simulink model "SkidSteeringControl"  (Simulink 8.9)
settings: Solver=VariableStepAuto  StartTime=0.0  StopTime=100  MaxStep=0.01  RelTol=1e-3
PreLoadFcn:
  | % Vehicle parameters
  | m = 1000;  % Vehicle mass
  | fR = 0.3;  % Front wheel radius
  | rR = 0.3;  % Rear wheel radius
  | J_front = 0.5;  % Front wheel moment of inertia
  | J_rear = 0.5;  % Rear wheel moment of inertia
  | J_engine = 0.01; % Engine moment of inertia
  | trans_ratio = 2.0;  % Transmission gear ratio
  | drive_ratio = 2.0;  % Final drive gear ratio
  | h = 0.5;   % Vehicle CG height above ground
  | 
  | % Aerodynamic load
  | cw = 0.34;  % Drag coefficient
  | rho = 1.18; % Air density
  | A_f = 1;    % Frontal area
  | 
  | 
  | %tire parameters
  | radiusWheel = 16*2.54/100;
  | inertiaLateral = 25*(radiusWheel)^2;
  | tireStiffness = 200000;
  | tireDamping = 1000;
StopFcn:
  | %%
  | close all;
  | figure;plot(disp_x,disp_y);grid on;axis('tight');
  | title('Vehicle Displacement Plot');
  | xlabel('Displacement X(m)');ylabel('Displacement Y(m)');
  | %%
  | figure;
  | subplot(2,1,1);
  | plot(desired_speedFL.time, desired_speedFL.signals.values,'g');grid on;hold on;
  | plot(desired_speedFR.time, desired_speedFR.signals.values,'b');grid on;
  | title('Desired Wheel Speed');
  | legend('Wheel Speed FL','Wheel Speed FR');
  | subplot(2,1,2);
  | plot(ref_speedFL.time, ref_speedFL.signals.values,'g');grid on;hold on;
  | plot(ref_speedFR.time, ref_speedFR.signals.values,'b');grid on;
  | title('Reference Wheel Speed(Slip Compensated)');
  | legend('Wheel Speed FL','Wheel Speed FR');
  | %%
  | figure;plot(yaw_rate.time,yaw_rate.signals.values);grid on;
  | title('Vehicle Yaw Rate');
  | xlabel('time(s)');ylabel('Yaw Rate(rad/s)');
  | %%
  | figure;
  | subplot(2,1,1);
  | plot(slip_WheelFL.time, slip_WheelFL.signals.values);grid on;
  | title('Wheel Slip Front Left');
  | xlabel('time(s)');ylabel('Slip Ratio');
  | subplot(2,1,2);
  | plot(slip_WheelFR.time, slip_WheelFR.signals.values);grid on;
  | title('Wheel Slip Front Right');
  | xlabel('time(s)');ylabel('Slip Ratio');
  | %%
  | figure;
  | subplot(2,1,1);
  | plot(torque_WheelFL.time, torque_WheelFL.signals.values);grid on;
  | title('Wheel Torque Front Left');
  | xlabel('time(s)');ylabel('Torque(Nm)');
  | subplot(2,1,2);
  | plot(torque_WheelFR.time, torque_WheelFR.signals.values);grid on;
  | title('Wheel Torque Front Right');
  | xlabel('time(s)');ylabel('Torque(Nm)');
libraries: nesl_utility x8, fl_lib x4, sdl_lib x4, simulink_extras x2, simulink x1
(part 2 of 2)

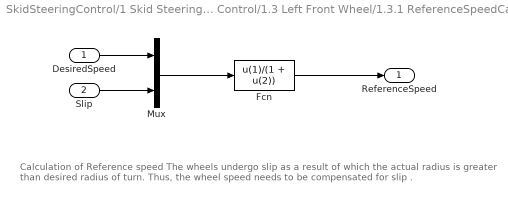
== system SkidSteeringControl/1 Skid Steering Control/1.3 Left Front Wheel/1.3.1 ReferenceSpeedCalcFR ==
  note: Calculation of Reference speed
      | The wheels undergo slip as a result of which the actual radius is greater than desired radius of turn.
      | Thus, the wheel speed needs to be compensated for slip
      | .
  DesiredSpeed : Inport
  "Slip " : Inport  Port=2
  Fcn : Fcn  Expr=u(1)/(1 + u(2))
  Mux : Mux  Inputs=2
  ReferenceSpeed : Outport
  wires:
  "Slip "/1 -> Mux/2
  Fcn/1 -> ReferenceSpeed/1
  DesiredSpeed/1 -> Mux/1
  Mux/1 -> Fcn/1

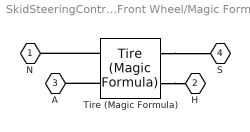
== system SkidSteeringControl/1 Skid Steering Control/1.3 Left Front Wheel/Magic Formula ==
  Tire (Magic Formula) : sdl_lib/Tires & Vehicles/Tire (Magic Formula)  parameterization=1  F_z1=3000 N  F_x1=3500 N  kappa1=10  B_m=10  C_m=1.9  D_m=1  E_m=0.97  fz0=4e+3 N  p_Cx=1.685  p_Dx=[ 1.21 -0.037 ]  p_Ex=[ 0.344 0.095 -0.02 0 ]  p_Kx=[ 21.51 -0.163 0.245 ]  p_Hx=[ -0.002 0.002 ]  p_Vx=[ 0 0 ]  v_tr_thr=0.1 m/s  r_e=radiusWheel m  model_compliance=1  stiffness=tireStiffness N/m  damping=tireDamping N/(m/s)  model_inertia=1  inertia=inertiaLateral/2 kg*m^2  initial_velocity=0 rpm  model_resistance=1  resistance_model=1  coeff=0.015  p_tire=250e3 Pa  alpha=-0.003  beta=0.97  coeff_a=84e-4  coeff_b=6.2e-4 s/m  coeff_c=1.6e-4 s^2/m^2  v_thr=1e-3 m/s
      settings: SourceProductName=Simscape Driveline
  N : PMIOPort  Port=1  Side=Left
  H : PMIOPort  Port=2  Side=Left
  A : PMIOPort  Port=3  Side=Left
  S : PMIOPort  Port=4  Side=Right
  connections:
  Tire (Magic Formula)/LConn2 -- A/RConn1
  Tire (Magic Formula)/LConn1 -- N/RConn1
  Tire (Magic Formula)/RConn2 -- H/RConn1
  Tire (Magic Formula)/RConn1 -- S/RConn1

== system SkidSteeringControl/1 Skid Steering Control/1.3 Left Front Wheel/SlipOut ==
  PS-Simulink Converter : nesl_utility/PS-Simulink Converter  PhysicalDomain=network_engine_domain  SubClassName=ps_output  LeftPortType=input  RightPortType=output  PseudoPeriodic=off  Frequencies=[]  Unit=1  AffineConversion=off
  S : PMIOPort  Port=1  Side=Left
  Slip : Outport
  wires:
  PS-Simulink Converter/1 -> Slip/1
  connections:
  S/RConn1 -- PS-Simulink Converter/LConn1

== system SkidSteeringControl/1 Skid Steering Control/1.4 Right Front Wheel/1.4.1 ReferenceSpeedCalcFR ==
  note: Calculation of Reference speed
      | The wheels undergo slip as a result of which the actual radius is greater than desired radius of turn.
      | Thus, the wheel speed needs to be compensated for slip
      | .
  DesiredSpeed : Inport
  "Slip " : Inport  Port=2
  Fcn : Fcn  Expr=u(1)/(1 + u(2))
  Mux : Mux  Inputs=2
  ReferenceSpeed : Outport
  wires:
  "Slip "/1 -> Mux/2
  Fcn/1 -> ReferenceSpeed/1
  DesiredSpeed/1 -> Mux/1
  Mux/1 -> Fcn/1

== system SkidSteeringControl/1 Skid Steering Control/1.4 Right Front Wheel/Magic Formula ==
  Tire (Magic Formula) : sdl_lib/Tires & Vehicles/Tire (Magic Formula)  parameterization=1  F_z1=3000 N  F_x1=3500 N  kappa1=10  B_m=10  C_m=1.9  D_m=1  E_m=0.97  fz0=4e+3 N  p_Cx=1.685  p_Dx=[ 1.21 -0.037 ]  p_Ex=[ 0.344 0.095 -0.02 0 ]  p_Kx=[ 21.51 -0.163 0.245 ]  p_Hx=[ -0.002 0.002 ]  p_Vx=[ 0 0 ]  v_tr_thr=0.1 m/s  r_e=radiusWheel m  model_compliance=1  stiffness=tireStiffness N/m  damping=tireDamping N/(m/s)  model_inertia=1  inertia=inertiaLateral/2 kg*m^2  initial_velocity=0 rpm  model_resistance=1  resistance_model=1  coeff=0.015  p_tire=250e3 Pa  alpha=-0.003  beta=0.97  coeff_a=84e-4  coeff_b=6.2e-4 s/m  coeff_c=1.6e-4 s^2/m^2  v_thr=1e-3 m/s
      settings: SourceProductName=Simscape Driveline
  N : PMIOPort  Port=1  Side=Left
  H : PMIOPort  Port=2  Side=Left
  A : PMIOPort  Port=3  Side=Left
  S : PMIOPort  Port=4  Side=Right
  connections:
  Tire (Magic Formula)/LConn2 -- A/RConn1
  Tire (Magic Formula)/LConn1 -- N/RConn1
  Tire (Magic Formula)/RConn2 -- H/RConn1
  Tire (Magic Formula)/RConn1 -- S/RConn1

== system SkidSteeringControl/1 Skid Steering Control/1.4 Right Front Wheel/SlipOut ==
  PS-Simulink Converter : nesl_utility/PS-Simulink Converter  PhysicalDomain=network_engine_domain  SubClassName=ps_output  LeftPortType=input  RightPortType=output  PseudoPeriodic=off  Frequencies=[]  Unit=1  AffineConversion=off
  S : PMIOPort  Port=1  Side=Left
  Slip : Outport
  wires:
  PS-Simulink Converter/1 -> Slip/1
  connections:
  S/RConn1 -- PS-Simulink Converter/LConn1

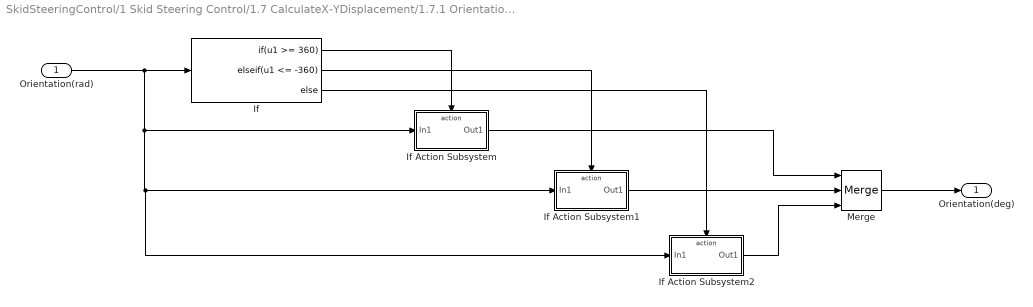
== system SkidSteeringControl/1 Skid Steering Control/1.7 CalculateX-YDisplacement/1.7.1 Orientation Calculation ==
  Orientation(rad) : Inport
  If : If  IfExpression=u1 >= 360  ElseIfExpressions=u1 <= -360
  If Action Subsystem : Subsystem  TreatAsAtomicUnit=on
  If Action Subsystem1 : Subsystem  TreatAsAtomicUnit=on
  If Action Subsystem2 : Subsystem  TreatAsAtomicUnit=on
  Merge : Merge  Inputs=3
  Orientation(deg) : Outport
  wires:
  If/3 -> If Action Subsystem2/Action
  If Action Subsystem2/1(Out1) -> Merge/3
  If/2 -> If Action Subsystem1/Action
  If/1 -> If Action Subsystem/Action
  Orientation(rad)/1 -> If Action Subsystem2/1(In1), If Action Subsystem1/1(In1), If Action Subsystem/1(In1), If/1
  Merge/1 -> Orientation(deg)/1
  If Action Subsystem1/1(Out1) -> Merge/2
  If Action Subsystem/1(Out1) -> Merge/1

== system SkidSteeringControl/1 Skid Steering Control/1.7 CalculateX-YDisplacement/1.7.1 Orientation Calculation/If Action Subsystem ==
  In1 : Inport
  Action Port : ActionPort  ActionType=then
  Fcn : Fcn  Expr=u(1) - floor(u(1)/360)*360
  Out1 : Outport
  wires:
  In1/1 -> Fcn/1
  Fcn/1 -> Out1/1

== system SkidSteeringControl/1 Skid Steering Control/1.7 CalculateX-YDisplacement/1.7.1 Orientation Calculation/If Action Subsystem1 ==
  In1 : Inport
  Action Port : ActionPort  ActionType=elseif
  Fcn : Fcn  Expr=floor(abs(u(1)/360))*360 + u(1)
  Out1 : Outport
  wires:
  In1/1 -> Fcn/1
  Fcn/1 -> Out1/1

== system SkidSteeringControl/1 Skid Steering Control/1.7 CalculateX-YDisplacement/1.7.1 Orientation Calculation/If Action Subsystem2 ==
  In1 : Inport
  Action Port : ActionPort  ActionType=else
  Out1 : Outport
  wires:
  In1/1 -> Out1/1
